simulink model "EE2_Observateur"  (R2012b)
settings: Solver=ode45  StartTime=0.0  StopTime=5  RelTol=1e-5
undefined symbols (not defined in the file or in its folder): EE0, EE1, EE2, obsver
settings Model: Creator=Lucien  LastModifiedBy=David
settings OptimizationCC: ExpressionDepthLimit=128
settings DebuggingCC: UnderspecifiedInitializationDetection=Simplified  MergeDetectMultiDrivingBlocksExec=error  SolverPrmCheckMsg=none  FrameProcessingCompatibilityMsg=error  StateNameClashWarn=none
settings CodeAppCC: CustomSymbolStrType=$N$R$M_T
settings GRTTargetCC: CodeReplacementLibrary=C89/C90 (ANSI)

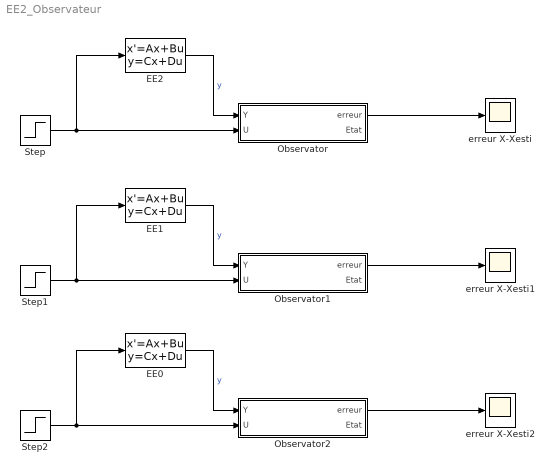
== system EE2_Observateur ==
  EE0 : StateSpace  A=EE0.ee.a  B=EE0.ee.b  C=EE0.ee.c  D=EE0.ee.d  X0=0
  EE1 : StateSpace  A=EE1.ee.a  B=EE1.ee.b  C=EE1.ee.c  D=EE1.ee.d  X0=0
  "EE2 " : StateSpace  A=EE2.ee.a  B=EE2.ee.b  C=EE2.ee.c  D=EE2.ee.d  X0=0
  Observator : Subsystem
  Observator1 : Subsystem
  Observator2 : Subsystem
  Step : Step  Time=0  SampleTime=0
  Step1 : Step  Time=0  SampleTime=0
  Step2 : Step  Time=0  SampleTime=0
  erreur X-Xesti : Scope
      settings: SaveName=Erreur_obsv_EE2
  erreur X-Xesti1 : Scope
      settings: SaveName=Erreur_obsv_EE1
  erreur X-Xesti2 : Scope
      settings: SaveName=Erreur_obsv_EE0
  wires:
  Observator/1(erreur) -> erreur X-Xesti/1
  "EE2 "/1 -> Observator/1("Y ")  "y"
  Step/1 -> "EE2 "/1, Observator/2(U)
  Observator1/1(erreur) -> erreur X-Xesti1/1
  EE1/1 -> Observator1/1("Y ")  "y"
  Step1/1 -> EE1/1, Observator1/2(U)
  Observator2/1(erreur) -> erreur X-Xesti2/1
  EE0/1 -> Observator2/1("Y ")  "y"
  Step2/1 -> EE0/1, Observator2/2(U)

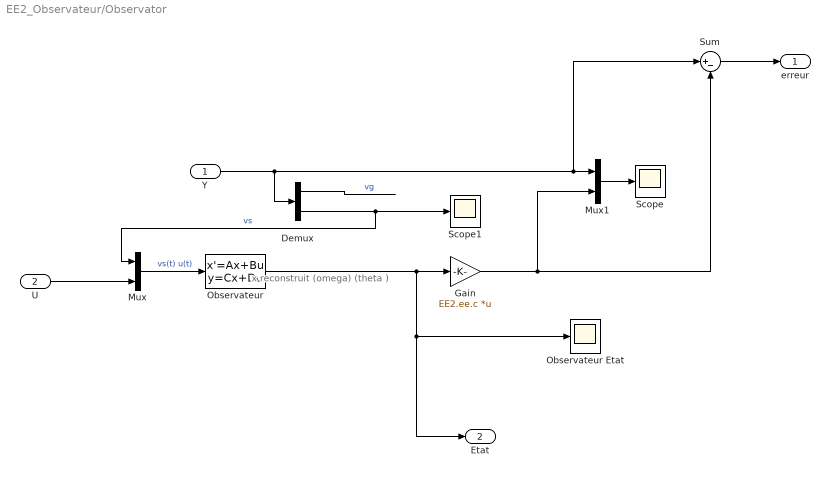
== system EE2_Observateur/Observator ==
  note: x reconstruit
      | (omega)
      | (theta   )
  "Y " : Inport
  U : Inport  Port=2
  Demux : Demux  Outputs=2
  Gain : Gain  Gain=EE2.ee.c  Multiplication=Matrix(K*u)
  Mux : Mux  Inputs=2
  Mux1 : Mux  Inputs=2
  "Observateur " : StateSpace  A=obsver.ee.a  B=obsver.ee.b  C=obsver.ee.c  D=obsver.ee.d  X0=0
  "Observateur Etat " : Scope
  Scope : Scope
      settings: YMin=-1  YMax=1
  Scope1 : Scope
      settings: YMin=16  YMax=30  SaveName=ScopeData2
  Sum : Sum  Inputs=|+-
  erreur : Outport
  "Etat " : Outport  Port=2
  wires:
  Mux1/1 -> Scope/1
  "Observateur "/1 -> "Etat "/1, "Observateur Etat "/1, Gain/1
  Demux/2 -> Mux/1, Scope1/1  "vs"
  Sum/1 -> erreur/1
  Demux/1 -> ?  "vg"
  "Y "/1 -> Sum/1, Mux1/1, Demux/1
  Mux/1 -> "Observateur "/1  "vs(t) u(t)"
  Gain/1 -> Mux1/2, Sum/2
  U/1 -> Mux/2

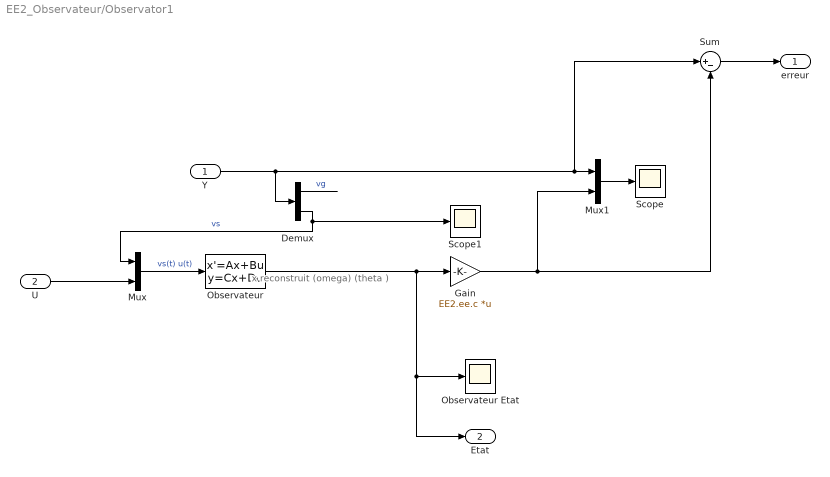
== system EE2_Observateur/Observator1 ==
  note: x reconstruit
      | (omega)
      | (theta   )
  "Y " : Inport
  U : Inport  Port=2
  Demux : Demux  Outputs=2
  Gain : Gain  Gain=EE2.ee.c  Multiplication=Matrix(K*u)
  Mux : Mux  Inputs=2
  Mux1 : Mux  Inputs=2
  "Observateur " : StateSpace  A=obsver.ee.a  B=obsver.ee.b  C=obsver.ee.c  D=obsver.ee.d  X0=0
  "Observateur Etat " : Scope
  Scope : Scope
  Scope1 : Scope
      settings: SaveName=ScopeData2
  Sum : Sum  Inputs=|+-
  erreur : Outport
  "Etat " : Outport  Port=2
  wires:
  Mux1/1 -> Scope/1
  "Observateur "/1 -> "Etat "/1, "Observateur Etat "/1, Gain/1
  Demux/2 -> Scope1/1, Mux/1  "vs"
  Sum/1 -> erreur/1
  Demux/1 -> ?  "vg"
  "Y "/1 -> Sum/1, Mux1/1, Demux/1
  Mux/1 -> "Observateur "/1  "vs(t) u(t)"
  Gain/1 -> Mux1/2, Sum/2
  U/1 -> Mux/2

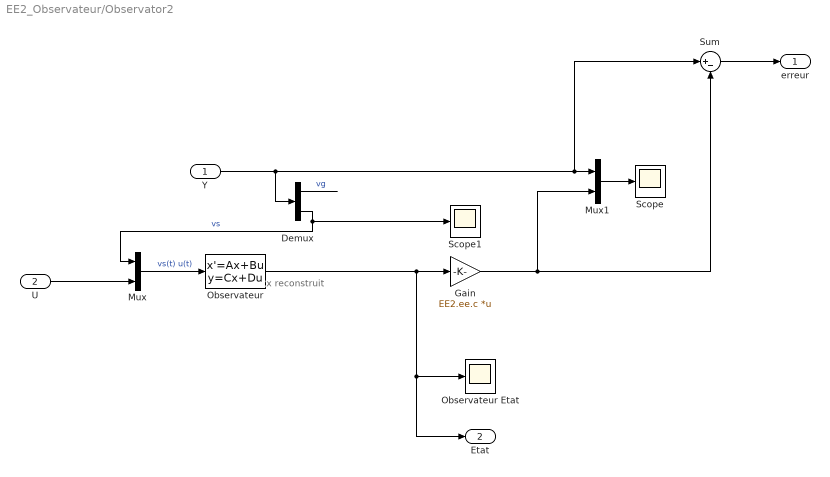
== system EE2_Observateur/Observator2 ==
  note: x reconstruit
  "Y " : Inport
  U : Inport  Port=2
  Demux : Demux  Outputs=2
  Gain : Gain  Gain=EE2.ee.c  Multiplication=Matrix(K*u)
  Mux : Mux  Inputs=2
  Mux1 : Mux  Inputs=2
  "Observateur " : StateSpace  A=obsver.ee.a  B=obsver.ee.b  C=obsver.ee.c  D=obsver.ee.d  X0=0
  "Observateur Etat " : Scope
  Scope : Scope
  Scope1 : Scope
      settings: SaveName=ScopeData2
  Sum : Sum  Inputs=|+-
  erreur : Outport
  "Etat " : Outport  Port=2
  wires:
  Mux1/1 -> Scope/1
  "Observateur "/1 -> "Etat "/1, "Observateur Etat "/1, Gain/1
  Demux/2 -> Scope1/1, Mux/1  "vs"
  Sum/1 -> erreur/1
  Demux/1 -> ?  "vg"
  "Y "/1 -> Sum/1, Mux1/1, Demux/1
  Mux/1 -> "Observateur "/1  "vs(t) u(t)"
  Gain/1 -> Mux1/2, Sum/2
  U/1 -> Mux/2
